simulink library "aerolibgravity2"  (R2020a)
settings: Solver=ode45  StartTime=0.0  StopTime=10.0  RelTol=1e-3
PostLoadFcn:
  | load_system('aerolibv1')
  | setsysloc('aerolibv1')
undefined symbols (not defined in the file or in its folder): aeroassertmsg, C, geoidgrid, ghCurrent, GM, latbp, lonbp, minYearCurrent, Newton, nMax10, nMax13, nMaxBetween, nMaxCurrent, R, Raphson, S, svCurrent, tabNMax10, tabNMax13, tabNMaxBetween
libraries: simulink x17, aerolibgravitysys x4
(part 4 of 4)

== system aerolibgravity2/International Geomagnetic Reference Field 12/Calculate Field/Compute magnetic vector in spherical coordinates/Compute magnetic vector in spherical coordinates/Compute normalized associated legendre polynomials and derivatives via recursion relations/If Subsystem/If Action Subsystem ==
  p_old : Inport
  q_old : Inport  Port=2
  clat : Inport  Port=3
  slat : Inport  Port=4
  n : Inport  Port=5
  m : Inport  Port=6
  cnt : Inport  Port=7
  Action Port : ActionPort  PropagateVarSize=During execution
  Math Function : Math  Operator=reciprocal  SignedPower=on  SaturateOnIntegerOverflow=on
  Product : Product  SaturateOnIntegerOverflow=on  OutDataTypeStr=Inherit: Same as first input
  Product1 : Product  Inputs=4  SaturateOnIntegerOverflow=on  OutDataTypeStr=Inherit: Same as first input
  Product2 : Product  Inputs=***  SaturateOnIntegerOverflow=on  OutDataTypeStr=Inherit: Same as first input
  Product3 : Product  SaturateOnIntegerOverflow=on  OutDataTypeStr=Inherit: Same as first input
  Selector : Selector  InputPortWidth=nPG  IndexOptions=Index vector (port)  Indices=[1 3]  OutputSizes=1
  Selector1 : Selector  InputPortWidth=nPG  IndexOptions=Index vector (port)  Indices=1  OutputSizes=1
  Sum : Sum  Inputs=|++  SaturateOnIntegerOverflow=on
  calculate index : Subsystem
  calculate mult : Subsystem
  p : Outport  VectorParamsAs1DForOutWhenUnconnected=off
  q : Outport  Port=2  VectorParamsAs1DForOutWhenUnconnected=off
  wires:
  Product3/1 -> q/1
  Math Function/1 -> Product2/1
  calculate mult/2(aa) -> Product3/1, Product1/4
  calculate mult/1(p_mult) -> Product1/3
  m/1 -> Math Function/1, calculate mult/1(m)
  cnt/1 -> calculate index/2(cnt)
  Product2/1 -> Sum/1
  slat/1 -> Product2/2
  Product1/1 -> p/1
  Selector/1 -> Product2/3, Product1/2
  Product/1 -> Sum/2
  Sum/1 -> Product3/2
  clat/1 -> Product1/1, Product/1
  Selector1/1 -> Product/2
  q_old/1 -> Selector1/1
  p_old/1 -> Selector/1
  calculate index/1(j) -> Selector1/2, Selector/2
  n/1 -> calculate index/1(n)

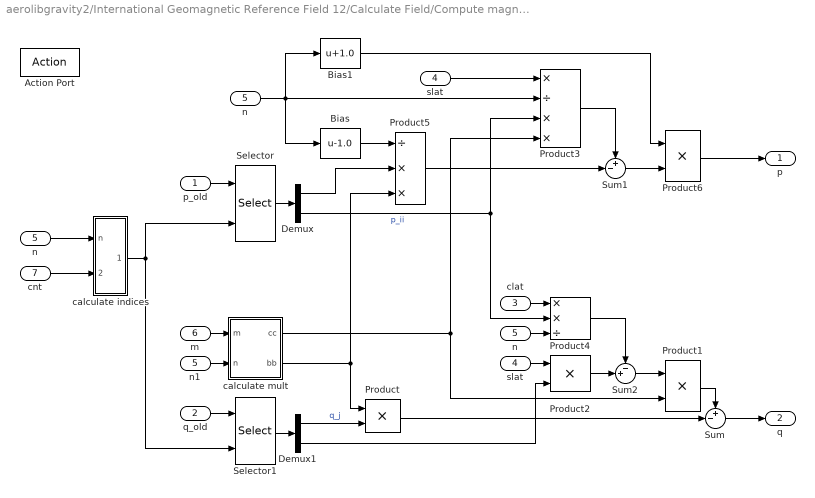
== system aerolibgravity2/International Geomagnetic Reference Field 12/Calculate Field/Compute magnetic vector in spherical coordinates/Compute magnetic vector in spherical coordinates/Compute normalized associated legendre polynomials and derivatives via recursion relations/If Subsystem/If Action Subsystem2 ==
  p_old : Inport
  q_old : Inport  Port=2
  clat : Inport  Port=3
  slat : Inport  Port=4
  n : Inport  Port=5
  m : Inport  Port=6
  cnt : Inport  Port=7
  Action Port : ActionPort  PropagateVarSize=During execution
  " n" : InportShadow  Port=5
  Bias : Bias  Bias=-1.0
  Bias1 : Bias  Bias=1.0
  Demux : Demux  Outputs=2
      settings: DisplayOption=none
  Demux1 : Demux  Outputs=2
      settings: DisplayOption=none
  Product{,1..2,6} (4 alike) : Product  SaturateOnIntegerOverflow=on  OutDataTypeStr=Inherit: Same as first input
  Product3 : Product  Inputs=*/**  SaturateOnIntegerOverflow=on  OutDataTypeStr=Inherit: Same as first input
  Product4 : Product  Inputs=**/  SaturateOnIntegerOverflow=on  OutDataTypeStr=Inherit: Same as first input
  Product5 : Product  Inputs=/**  SaturateOnIntegerOverflow=on  OutDataTypeStr=Inherit: Same as first input
  Selector : Selector  InputPortWidth=nPG  IndexOptions=Index vector (port)  Indices=[1 3]  OutputSizes=1
  Selector1 : Selector  InputPortWidth=nPG  IndexOptions=Index vector (port)  Indices=[1 3]  OutputSizes=1
  Sum : Sum  Inputs=+-|  SaturateOnIntegerOverflow=on
  Sum1 : Sum  Inputs=+-|  SaturateOnIntegerOverflow=on
  Sum2 : Sum  Inputs=-+|  SaturateOnIntegerOverflow=on
  calculate indices : Subsystem
  calculate mult : Subsystem
  "n " : InportShadow  Port=5
  n1 : InportShadow  Port=5
  "slat " : InportShadow  Port=4
  p : Outport  VectorParamsAs1DForOutWhenUnconnected=off
  q : Outport  Port=2  VectorParamsAs1DForOutWhenUnconnected=off
  wires:
  n1/1 -> calculate mult/2(n)
  Product6/1 -> p/1
  Bias1/1 -> Product6/1
  Product3/1 -> Sum1/1
  Bias/1 -> Product5/1
  Product5/1 -> Sum1/2
  Demux/1 -> Product5/2
  " n"/1 -> Product3/2, Bias1/1, Bias/1
  "slat "/1 -> Product2/1
  Demux1/2 -> Product2/2
  Product2/1 -> Sum2/2
  calculate mult/1(cc) -> Product3/4, Product1/2
  Product1/1 -> Sum/1
  Sum2/1 -> Product1/1
  m/1 -> calculate mult/1(m)
  Product4/1 -> Sum2/1
  "n "/1 -> Product4/3
  calculate mult/2(bb) -> Product5/3, Product/1
  cnt/1 -> calculate indices/2(cnt)
  Sum1/1 -> Product6/2
  Demux/2 -> Product3/3, Product4/2  "p_ii"
  Sum/1 -> q/1
  Demux1/1 -> Product/2  "q_j"
  Selector/1 -> Demux/1
  clat/1 -> Product4/1
  Product/1 -> Sum/2
  slat/1 -> Product3/1
  Selector1/1 -> Demux1/1
  q_old/1 -> Selector1/1
  p_old/1 -> Selector/1
  calculate indices/1(j,ii) -> Selector1/2, Selector/2
  n/1 -> calculate indices/1(n)

== system aerolibgravity2/International Geomagnetic Reference Field 12/Calculate Field/Compute magnetic vector in spherical coordinates/Compute magnetic vector in spherical coordinates/Compute normalized associated legendre polynomials and derivatives via recursion relations/If Subsystem/p(1:4) ==
  bus : Inport
  Bus Selector2 : BusSelector  OutputSignals=slat,clat,slat,slat,clat
  Constant : Constant  Value=3
  Constant1 : Constant  Value=1.5
  Gain : Gain  Gain=4.5
  Gain1 : Gain  Gain=2
  Gain2 : Gain  Gain=2
  Product3 : Product  Inputs=4  SaturateOnIntegerOverflow=on  OutDataTypeStr=Inherit: Same as first input
  Product4 : Product  SaturateOnIntegerOverflow=on  OutDataTypeStr=Inherit: Same as first input
  Sqrt : Sqrt  SaturateOnIntegerOverflow=on
  Sum2 : Sum  Inputs=-+|  SaturateOnIntegerOverflow=on
  Vector Concatenate : Concatenate  NumInputs=4
  p(1:4) : Outport  VectorParamsAs1DForOutWhenUnconnected=off
  wires:
  Vector Concatenate/1 -> p(1:4)/1
  bus/1 -> Bus Selector2/1
  Constant/1 -> Sqrt/1, Product3/3
  Product3/1 -> Vector Concatenate/4
  Sqrt/1 -> Product3/4
  Bus Selector2/5 -> Product3/2  "<clat>"
  Gain/1 -> Sum2/2
  Sum2/1 -> Vector Concatenate/3
  Product4/1 -> Gain/1
  Gain1/1 -> Vector Concatenate/1
  Gain2/1 -> Vector Concatenate/2
  Constant1/1 -> Sum2/1
  Bus Selector2/1 -> Gain1/1  "<slat>"
  Bus Selector2/2 -> Gain2/1  "<clat>"
  Bus Selector2/4 -> Product3/1  "<slat>"
  Bus Selector2/3 -> Product4/2, Product4/1  "<slat>"

== system aerolibgravity2/International Geomagnetic Reference Field 12/Calculate Field/Compute magnetic vector in spherical coordinates/Compute magnetic vector in spherical coordinates/Compute normalized associated legendre polynomials and derivatives via recursion relations/If Subsystem/q(1:4) ==
  bus : Inport
  Bus Selector2 : BusSelector  OutputSignals=clat,slat,slat,clat,slat,clat
  Constant : Constant  Value=3
  Gain : Gain  Gain=3
  Product{1..4} (4 alike) : Product  SaturateOnIntegerOverflow=on  OutDataTypeStr=Inherit: Same as first input
  Sqrt : Sqrt  SaturateOnIntegerOverflow=on
  Sum1 : Sum  Inputs=+-|  SaturateOnIntegerOverflow=on
  Unary Minus : UnaryMinus
  Unary Minus1 : UnaryMinus
  Vector Concatenate : Concatenate  NumInputs=4
  q(1:4) : Outport  VectorParamsAs1DForOutWhenUnconnected=off
  wires:
  Unary Minus/1 -> Vector Concatenate/1
  Bus Selector2/3 -> Product4/1  "<slat>"
  Bus Selector2/4 -> Product4/2  "<clat>"
  Product4/1 -> Gain/1
  Unary Minus1/1 -> Vector Concatenate/3
  Gain/1 -> Unary Minus1/1
  Bus Selector2/5 -> Product1/2, Product1/1  "<slat>"
  Bus Selector2/6 -> Product2/1, Product2/2  "<clat>"
  Product2/1 -> Sum1/2
  Product1/1 -> Sum1/1
  Sum1/1 -> Product3/1
  Sqrt/1 -> Product3/2
  Product3/1 -> Vector Concatenate/4
  Constant/1 -> Sqrt/1
  bus/1 -> Bus Selector2/1
  Vector Concatenate/1 -> q(1:4)/1
  Bus Selector2/1 -> Unary Minus/1  "<clat>"
  Bus Selector2/2 -> Vector Concatenate/2  "<slat>"

== system aerolibgravity2/International Geomagnetic Reference Field 12/Calculate Field/Compute magnetic vector in spherical coordinates/Compute magnetic vector in spherical coordinates/Compute normalized associated legendre polynomials and derivatives via recursion relations/If Subsystem/If Action Subsystem/calculate index ==
  n : Inport
  cnt : Inport  Port=2
  Constant : Constant  OutDataTypeStr=Inherit: Inherit via back propagation
  Sum2 : Sum  Inputs=+--  SaturateOnIntegerOverflow=on
  j : Outport  VectorParamsAs1DForOutWhenUnconnected=off
  wires:
  cnt/1 -> Sum2/1
  Constant/1 -> Sum2/3
  n/1 -> Sum2/2
  Sum2/1 -> j/1

== system aerolibgravity2/International Geomagnetic Reference Field 12/Calculate Field/Compute magnetic vector in spherical coordinates/Compute magnetic vector in spherical coordinates/Compute normalized associated legendre polynomials and derivatives via recursion relations/If Subsystem/If Action Subsystem/calculate mult ==
  m : Inport
  Constant : Constant  OutDataTypeStr=Inherit: Inherit via back propagation
  Constant1 : Constant  Value=0.5  OutDataTypeStr=Inherit: Inherit via back propagation
  Constant2 : Constant  OutDataTypeStr=Inherit: Inherit via back propagation
  Math Function : Math  Operator=reciprocal  SignedPower=on  SaturateOnIntegerOverflow=on
  Product1 : Product  Inputs=*/  SaturateOnIntegerOverflow=on  OutDataTypeStr=Inherit: Same as first input
  Sqrt : Sqrt  SaturateOnIntegerOverflow=on
  Sum1 : Sum  Inputs=|++  SaturateOnIntegerOverflow=on
  Sum2 : Sum  Inputs=+-|  SaturateOnIntegerOverflow=on
  p_mult : Outport  VectorParamsAs1DForOutWhenUnconnected=off
  aa : Outport  Port=2  VectorParamsAs1DForOutWhenUnconnected=off
  wires:
  Sum1/1 -> p_mult/1
  Constant2/1 -> Sum1/2
  Math Function/1 -> Sum1/1
  Sqrt/1 -> aa/1
  Product1/1 -> Sum2/2
  m/1 -> Math Function/1, Product1/2
  Constant1/1 -> Product1/1
  Constant/1 -> Sum2/1
  Sum2/1 -> Sqrt/1

== system aerolibgravity2/International Geomagnetic Reference Field 12/Calculate Field/Compute magnetic vector in spherical coordinates/Compute magnetic vector in spherical coordinates/Compute normalized associated legendre polynomials and derivatives via recursion relations/If Subsystem/If Action Subsystem2/calculate indices ==
  n : Inport
  cnt : Inport  Port=2
  Constant1 : Constant  OutDataTypeStr=Inherit: Inherit via back propagation
  Gain : Gain  Gain=2  SaturateOnIntegerOverflow=on  OutDataTypeStr=Inherit: Same as input  ParamDataTypeStr=Inherit: Same as input
  Mux : Mux  Inputs=2
  Sum1 : Sum  Inputs=+-+  SaturateOnIntegerOverflow=on
  Sum3 : Sum  Inputs=|-+  SaturateOnIntegerOverflow=on
  j,ii : Outport  VectorParamsAs1DForOutWhenUnconnected=off
  wires:
  Gain/1 -> Sum1/2
  Mux/1 -> j,ii/1
  Sum3/1 -> Mux/2
  cnt/1 -> Sum1/1, Sum3/2
  Constant1/1 -> Sum1/3
  Sum1/1 -> Mux/1
  n/1 -> Gain/1, Sum3/1

== system aerolibgravity2/International Geomagnetic Reference Field 12/Calculate Field/Compute magnetic vector in spherical coordinates/Compute magnetic vector in spherical coordinates/Compute normalized associated legendre polynomials and derivatives via recursion relations/If Subsystem/If Action Subsystem2/calculate mult ==
  m : Inport
  n : Inport  Port=2
  " n" : InportShadow  Port=2
  Bias : Bias  Bias=-1.0
  Constant2 : Constant  OutDataTypeStr=Inherit: Inherit via back propagation
  Gain : Gain  Gain=2  SaturateOnIntegerOverflow=on  OutDataTypeStr=Inherit: Same as input  ParamDataTypeStr=Inherit: Same as input
  Product1 : Product  SaturateOnIntegerOverflow=on  OutDataTypeStr=Inherit: Same as first input
  Product2 : Product  SaturateOnIntegerOverflow=on  OutDataTypeStr=Inherit: Same as first input
  Product3 : Product  Inputs=*/  SaturateOnIntegerOverflow=on  OutDataTypeStr=Inherit: Same as first input
  Product4 : Product  Inputs=/*  SaturateOnIntegerOverflow=on  OutDataTypeStr=Inherit: Same as first input
  Product5 : Product  SaturateOnIntegerOverflow=on  OutDataTypeStr=Inherit: Same as first input
  Sqrt : Sqrt  SaturateOnIntegerOverflow=on
  Sqrt1 : Sqrt  SaturateOnIntegerOverflow=on
  Sum1 : Sum  Inputs=|+-  SaturateOnIntegerOverflow=on
  Sum2 : Sum  Inputs=-+|  SaturateOnIntegerOverflow=on
  Sum3 : Sum  Inputs=+-|  SaturateOnIntegerOverflow=on
  "n " : InportShadow  Port=2
  cc : Outport  VectorParamsAs1DForOutWhenUnconnected=off
  bb : Outport  Port=2  VectorParamsAs1DForOutWhenUnconnected=off
  wires:
  " n"/1 -> Bias/1
  Bias/1 -> Product5/1, Product5/2
  Product5/1 -> Sum3/1
  Product2/1 -> Sum2/2
  Product1/1 -> Sum3/2, Sum2/1
  Sum3/1 -> Sqrt1/1
  Product4/1 -> cc/1
  "n "/1 -> Gain/1
  Product3/1 -> bb/1
  Sqrt1/1 -> Product3/1
  n/1 -> Product2/2, Product2/1
  Sum2/1 -> Sqrt/1
  m/1 -> Product1/1, Product1/2
  Sqrt/1 -> Product4/1, Product3/2
  Gain/1 -> Sum1/1
  Constant2/1 -> Sum1/2
  Sum1/1 -> Product4/2
